simulink model "updated_target_driver_2026"  (R2024b)
settings: Solver=VariableStepAuto  StartTime=0.0  StopTime=10.0  RelTol=1e-3
values from neighbouring files (symbols this model uses):
  A = gamma_2*gamma_3*Thrust_desired    [force2voltage.m]
  a2_lb = -0.25    [target_driver_setup_2022_Ctrl_V_2_4.m]    (also in target_driver_setup_2022_Ctrl_V_2_4_geometric.m; target_driver_setup_mpc_12msdelay.m; target_driver_setup_mpc_andWLQP.m)
  a2_openloop = -0    (= 0)    [target_driver_setup_2022_Ctrl_V_2_4.m]    (also in target_driver_setup_2022_Ctrl_V_2_4_geometric.m; target_driver_setup_mpc_12msdelay.m; target_driver_setup_mpc_andWLQP.m)
  a2_ub = 0.25    [target_driver_setup_2022_Ctrl_V_2_4.m]    (also in target_driver_setup_2022_Ctrl_V_2_4_geometric.m; target_driver_setup_mpc_12msdelay.m; target_driver_setup_mpc_andWLQP.m)
  adaptive_flag = 0    [target_driver_setup_2022_Ctrl_V_2_4.m]    (also in target_driver_setup_2022_Ctrl_V_2_4_geometric.m; target_driver_setup_mpc_12msdelay.m = 1; target_driver_setup_mpc_andWLQP.m = 1)
  adaptive_gain = [gamma_adaptive, adaptive_roll_limit, adaptive_pitch_limit, adaptive_yaw_limit, c_2_adaptive, gamma_lateral_adaptive, adaptive_x_limit, adaptive_y_limit, adaptive_z_limit, c_1_adaptive]    [target_driver_setup_2022_Ctrl_V_2_4.m]    (also in target_driver_setup_2022_Ctrl_V_2_4_geometric.m; target_driver_setup_mpc_12msdelay.m; target_driver_setup_mpc_andWLQP.m)
  adaptive_lateral_flag = 0    [target_driver_setup_2022_Ctrl_V_2_4.m]    (also in target_driver_setup_2022_Ctrl_V_2_4_geometric.m; target_driver_setup_mpc_12msdelay.m = 1; target_driver_setup_mpc_andWLQP.m = 1)
  adaptive_pitch_init = 0    [target_driver_setup_2022_Ctrl_V_2_4.m]    (also in target_driver_setup_2022_Ctrl_V_2_4_geometric.m; target_driver_setup_mpc_12msdelay.m; target_driver_setup_mpc_andWLQP.m)
  adaptive_pitch_limit = 0.1/(scale^2)    (= 1e-07)    [target_driver_setup_2022_Ctrl_V_2_4.m]    (also in target_driver_setup_2022_Ctrl_V_2_4_geometric.m = 3e-07; target_driver_setup_mpc_12msdelay.m; target_driver_setup_mpc_andWLQP.m)
  adaptive_pitch_limit_low = -adaptive_pitch_limit    (= -1e-07)    [target_driver_setup_2022_Ctrl_V_2_4.m]    (also in target_driver_setup_2022_Ctrl_V_2_4_geometric.m = -3e-07; target_driver_setup_mpc_12msdelay.m; target_driver_setup_mpc_andWLQP.m)
  adaptive_roll_init = 0    [target_driver_setup_2022_Ctrl_V_2_4.m]    (also in target_driver_setup_2022_Ctrl_V_2_4_geometric.m; target_driver_setup_mpc_12msdelay.m; target_driver_setup_mpc_andWLQP.m)
  adaptive_roll_limit = 0.3/(scale^2)    (= 3e-07)    [target_driver_setup_2022_Ctrl_V_2_4.m]    (also in target_driver_setup_2022_Ctrl_V_2_4_geometric.m; target_driver_setup_mpc_12msdelay.m; target_driver_setup_mpc_andWLQP.m)
  adaptive_roll_limit_low = -adaptive_roll_limit    (= -3e-07)    [target_driver_setup_2022_Ctrl_V_2_4.m]    (also in target_driver_setup_2022_Ctrl_V_2_4_geometric.m; target_driver_setup_mpc_12msdelay.m; target_driver_setup_mpc_andWLQP.m)
  adaptive_x_init = 0    [target_driver_setup_2022_Ctrl_V_2_4.m]    (also in target_driver_setup_2022_Ctrl_V_2_4_geometric.m; target_driver_setup_mpc_12msdelay.m; target_driver_setup_mpc_andWLQP.m)
  adaptive_x_limit = 0.15/(scale)    (= 0.00015)    [target_driver_setup_2022_Ctrl_V_2_4.m]    (also in target_driver_setup_2022_Ctrl_V_2_4_geometric.m = 7.5e-05; target_driver_setup_mpc_12msdelay.m; target_driver_setup_mpc_andWLQP.m)
  adaptive_x_limit_low = -adaptive_x_limit    (= -0.00015)    [target_driver_setup_2022_Ctrl_V_2_4.m]    (also in target_driver_setup_2022_Ctrl_V_2_4_geometric.m = -7.5e-05; target_driver_setup_mpc_12msdelay.m; target_driver_setup_mpc_andWLQP.m)
  adaptive_y_init = 0    [target_driver_setup_2022_Ctrl_V_2_4.m]    (also in target_driver_setup_2022_Ctrl_V_2_4_geometric.m; target_driver_setup_mpc_12msdelay.m; target_driver_setup_mpc_andWLQP.m)
  adaptive_y_limit = 0.15/(scale)    (= 0.00015)    [target_driver_setup_2022_Ctrl_V_2_4.m]    (also in target_driver_setup_2022_Ctrl_V_2_4_geometric.m = 7.5e-05; target_driver_setup_mpc_12msdelay.m; target_driver_setup_mpc_andWLQP.m)
  adaptive_y_limit_low = -adaptive_y_limit    (= -0.00015)    [target_driver_setup_2022_Ctrl_V_2_4.m]    (also in target_driver_setup_2022_Ctrl_V_2_4_geometric.m = -7.5e-05; target_driver_setup_mpc_12msdelay.m; target_driver_setup_mpc_andWLQP.m)
  adaptive_yaw_init = 0    [target_driver_setup_2022_Ctrl_V_2_4.m]    (also in target_driver_setup_2022_Ctrl_V_2_4_geometric.m; target_driver_setup_mpc_12msdelay.m; target_driver_setup_mpc_andWLQP.m)
  adaptive_yaw_limit = 0.035/(scale^2)    (= 3.5e-08)    [target_driver_setup_2022_Ctrl_V_2_4.m]    (also in target_driver_setup_2022_Ctrl_V_2_4_geometric.m; target_driver_setup_mpc_12msdelay.m; target_driver_setup_mpc_andWLQP.m)
  adaptive_yaw_limit_low = -adaptive_yaw_limit    (= -3.5e-08)    [target_driver_setup_2022_Ctrl_V_2_4.m]    (also in target_driver_setup_2022_Ctrl_V_2_4_geometric.m; target_driver_setup_mpc_12msdelay.m; target_driver_setup_mpc_andWLQP.m)
  adaptive_z_init = 0/scale    (= 0)    [target_driver_setup_2022_Ctrl_V_2_4.m]    (also in target_driver_setup_2022_Ctrl_V_2_4_geometric.m; target_driver_setup_mpc_12msdelay.m; target_driver_setup_mpc_andWLQP.m)
  adaptive_z_limit = 0.20/(scale)    (= 0.0002)    [target_driver_setup_2022_Ctrl_V_2_4.m]    (also in target_driver_setup_2022_Ctrl_V_2_4_geometric.m = 0.0008; target_driver_setup_mpc_12msdelay.m = 0.0008; target_driver_setup_mpc_andWLQP.m = 0.0008)
  adaptive_z_limit_low = -adaptive_z_limit/1    (= -0.0002)    [target_driver_setup_2022_Ctrl_V_2_4.m]    (also in target_driver_setup_2022_Ctrl_V_2_4_geometric.m = -0.0008; target_driver_setup_mpc_12msdelay.m = -0.0008; target_driver_setup_mpc_andWLQP.m = -0.0008)
  att_s = 500    [target_driver_setup_2022_Ctrl_V_2_4.m]    (also in target_driver_setup_2022_Ctrl_V_2_4_geometric.m; target_driver_setup_mpc_12msdelay.m; target_driver_setup_mpc_andWLQP.m)
  b_1_d_desired = [1,0,0]    [target_driver_setup_2022_Ctrl_V_2_4.m]    (also in target_driver_setup_2022_Ctrl_V_2_4_geometric.m; target_driver_setup_mpc_12msdelay.m; target_driver_setup_mpc_andWLQP.m)
  closedloop_flag = 1    [target_driver_setup_2022_Ctrl_V_2_4.m]    (also in target_driver_setup_2022_Ctrl_V_2_4_geometric.m = 0; target_driver_setup_mpc_12msdelay.m = 0; target_driver_setup_mpc_andWLQP.m = 0)
  control_gain = [k_x,k_v, k_R, k_Omega, k_z, k_vz, k_Rx]    [target_driver_setup_2022_Ctrl_V_2_4.m]    (also in target_driver_setup_2022_Ctrl_V_2_4_geometric.m = [k_x,k_v,k_R,k_Omega_pitch,k_Omega_roll,k_z,k_vz,k_Rx]; target_driver_setup_mpc_12msdelay.m = [k_x, k_v, k_R, k_Omega, k_z, k_vz, k_Rx,                  k; target_driver_setup_mpc_andWLQP.m = [k_x, k_v, k_R, k_Omega, k_z, k_vz, k_Rx,                  k)
  delay = delay-vicon_sample_cycle/2    [target_driver_setup_2022_Ctrl_V_2_4.m]    (also in target_driver_setup_2022_Ctrl_V_2_4_geometric.m; target_driver_setup_mpc_12msdelay.m; target_driver_setup_mpc_andWLQP.m)
  drv_amp = abs((vleft_p2p-vright_p2p))/2+min(vleft_p2p,vright_p2p)    [Wing_traj_to_Voltage.m]    (also in force2voltage.m; target_driver_setup_2022_Ctrl_V_2_4.m = 300; target_driver_setup_2022_Ctrl_V_2_4_geometric.m = 110; target_driver_setup_mpc_12msdelay.m = 150)
  drv_bias = max_drv_bias    (= 300)    [target_driver_setup_2022_Ctrl_V_2_4.m]    (also in target_driver_setup_2022_Ctrl_V_2_4_geometric.m = 200; target_driver_setup_mpc_12msdelay.m = 200; target_driver_setup_mpc_andWLQP.m = 200)
  drv_pitch_left = vleft_pitch    [Wing_traj_to_Voltage.m]    (also in force2voltage.m = 0; target_driver_setup_2022_Ctrl_V_2_4.m = 0; target_driver_setup_2022_Ctrl_V_2_4_geometric.m = 9.05; target_driver_setup_mpc_12msdelay.m = 9.05)
  drv_pitch_right = vright_pitch    [Wing_traj_to_Voltage.m]    (also in force2voltage.m = 0; target_driver_setup_2022_Ctrl_V_2_4.m = 0; target_driver_setup_2022_Ctrl_V_2_4_geometric.m = 9.05; target_driver_setup_mpc_12msdelay.m = 9.05)
  drv_roll = (vleft_p2p-vright_p2p)/4    [Wing_traj_to_Voltage.m]    (also in force2voltage.m; target_driver_setup_2022_Ctrl_V_2_4.m = 0; target_driver_setup_2022_Ctrl_V_2_4_geometric.m = -0.001; target_driver_setup_mpc_12msdelay.m = -0.001)
  f_fin = f    (= 180)    [target_driver_setup_2022_Ctrl_V_2_4.m]    (also in target_driver_setup_2022_Ctrl_V_2_4_geometric.m = 155; target_driver_setup_mpc_12msdelay.m = 155; target_driver_setup_mpc_andWLQP.m = 155)
  f_int = f    (= 180)    [target_driver_setup_2022_Ctrl_V_2_4.m]    (also in target_driver_setup_2022_Ctrl_V_2_4_geometric.m = 155; target_driver_setup_mpc_12msdelay.m = 155; target_driver_setup_mpc_andWLQP.m = 155)
  g = 9.8    [target_driver_setup_2022_Ctrl_V_2_4.m]    (also in target_driver_setup_2022_Ctrl_V_2_4_geometric.m; target_driver_setup_mpc_12msdelay.m; target_driver_setup_mpc_andWLQP.m = 9.81; test_full_attitude_mpc.m = 9.81)
  I_moment_vec = [Ixx, Iyy, Izz]    [target_driver_setup_2022_Ctrl_V_2_4.m]    (also in target_driver_setup_2022_Ctrl_V_2_4_geometric.m; target_driver_setup_mpc_12msdelay.m; target_driver_setup_mpc_andWLQP.m)
  landing_flag = 0    [target_driver_setup_2022_Ctrl_V_2_4.m]    (also in target_driver_setup_2022_Ctrl_V_2_4_geometric.m; target_driver_setup_mpc_12msdelay.m; target_driver_setup_mpc_andWLQP.m)
  landing_parameter = [start_delay+T,transition_rate, rising_time, falling_time, landing_rising_time, landing_z_decrease, landing_y_decrease, landing_x_decrease]    [target_driver_setup_2022_Ctrl_V_2_4.m]    (also in target_driver_setup_2022_Ctrl_V_2_4_geometric.m; target_driver_setup_mpc_12msdelay.m; target_driver_setup_mpc_andWLQP.m)
  low_bound = -8    [target_driver_setup_2022_Ctrl_V_2_4.m]    (also in target_driver_setup_2022_Ctrl_V_2_4_geometric.m = -5; target_driver_setup_mpc_12msdelay.m = -10; target_driver_setup_mpc_andWLQP.m = -10)
  low_bound_eR = -0.8    [target_driver_setup_2022_Ctrl_V_2_4.m]    (also in target_driver_setup_2022_Ctrl_V_2_4_geometric.m = -1.2; target_driver_setup_mpc_12msdelay.m = -1.2; target_driver_setup_mpc_andWLQP.m = -1.2)
  low_bound_vx = -0.5    [target_driver_setup_2022_Ctrl_V_2_4.m]    (also in target_driver_setup_2022_Ctrl_V_2_4_geometric.m; target_driver_setup_mpc_12msdelay.m; target_driver_setup_mpc_andWLQP.m)
  low_bound_vy = -0.5    [target_driver_setup_2022_Ctrl_V_2_4.m]    (also in target_driver_setup_2022_Ctrl_V_2_4_geometric.m; target_driver_setup_mpc_12msdelay.m; target_driver_setup_mpc_andWLQP.m)
  low_bound_vz = -0.5    [target_driver_setup_2022_Ctrl_V_2_4.m]    (also in target_driver_setup_2022_Ctrl_V_2_4_geometric.m; target_driver_setup_mpc_12msdelay.m; target_driver_setup_mpc_andWLQP.m)
  low_bound_x = -0.06    [target_driver_setup_2022_Ctrl_V_2_4.m]    (also in target_driver_setup_2022_Ctrl_V_2_4_geometric.m = -0.1; target_driver_setup_mpc_12msdelay.m = -0.6; target_driver_setup_mpc_andWLQP.m = -0.6)
  low_bound_y = -0.06    [target_driver_setup_2022_Ctrl_V_2_4.m]    (also in target_driver_setup_2022_Ctrl_V_2_4_geometric.m; target_driver_setup_mpc_12msdelay.m = -0.6; target_driver_setup_mpc_andWLQP.m = -0.6)
  low_bound_z = -0.04    [target_driver_setup_2022_Ctrl_V_2_4.m]    (also in target_driver_setup_2022_Ctrl_V_2_4_geometric.m; target_driver_setup_mpc_12msdelay.m = -0.1; target_driver_setup_mpc_andWLQP.m = -0.1)
  m = t <= t_zoom    [plot_roll_torque_cmd_vs_actual.m]    (also in plot_roll_torque_cmd_vs_actual_flightlog.m = t >= t0 & t <= t1; target_driver_setup_2022_Ctrl_V_2_4.m = 0.000124; target_driver_setup_2022_Ctrl_V_2_4_geometric.m = 8.5655e-05; target_driver_setup_mpc_12msdelay.m = 8.5655e-05)
  params_vec = [params_opt.delta_1, params_opt.delta_2, params_opt.delta_3,      params_opt.gamma_1, params_opt.gamma_2_1, params_opt.gamma_3,      params_opt.eta, params_opt.nu, params_opt.mu]'    [force2voltage_tuningSandbox.m]    (also in target_driver_setup_2022_Ctrl_V_2_4.m = [params_opt.delta_1, params_opt.delta_2, params_opt.delta_3,; target_driver_setup_2022_Ctrl_V_2_4_geometric.m = [params_opt.delta_1, params_opt.delta_2, params_opt.delta_3,; target_driver_setup_mpc_12msdelay.m = [params_opt.delta_1, params_opt.delta_2, params_opt.delta_3,; target_driver_setup_mpc_andWLQP.m = [params_opt.delta_1, params_opt.delta_2, params_opt.delta_3,)
  phase = 0    [target_driver_setup_2022_Ctrl_V_2_4.m]    (also in target_driver_setup_2022_Ctrl_V_2_4_geometric.m; target_driver_setup_mpc_12msdelay.m; target_driver_setup_mpc_andWLQP.m)
  r_desired = [default_x, default_y,z_desired]    [target_driver_setup_2022_Ctrl_V_2_4.m]    (also in target_driver_setup_2022_Ctrl_V_2_4_geometric.m; target_driver_setup_mpc_12msdelay.m; target_driver_setup_mpc_andWLQP.m)
  roll_offset_angle = 0    [target_driver_setup_2022_Ctrl_V_2_4.m]    (also in target_driver_setup_2022_Ctrl_V_2_4_geometric.m; target_driver_setup_mpc_12msdelay.m; target_driver_setup_mpc_andWLQP.m)
  running_time = start_delay+total_T    (= 9)    [target_driver_setup_2022_Ctrl_V_2_4.m]    (also in target_driver_setup_2022_Ctrl_V_2_4_geometric.m = 10; target_driver_setup_mpc_12msdelay.m = 0.5; target_driver_setup_mpc_andWLQP.m = 10)
  running_time_control = start_delay_control+total_T+0.0    (= 7.1)    [target_driver_setup_2022_Ctrl_V_2_4.m]    (also in target_driver_setup_2022_Ctrl_V_2_4_geometric.m = 10; target_driver_setup_mpc_12msdelay.m = 0.5; target_driver_setup_mpc_andWLQP.m = 10)
  start_delay = 2.0    (= 2)    [target_driver_setup_2022_Ctrl_V_2_4.m]    (also in target_driver_setup_2022_Ctrl_V_2_4_geometric.m = 0; target_driver_setup_mpc_12msdelay.m = 0; target_driver_setup_mpc_andWLQP.m = 0)
  start_delay_control = start_delay + ramp_delay    (= 0.1)    [target_driver_setup_2022_Ctrl_V_2_4.m]    (also in target_driver_setup_2022_Ctrl_V_2_4_geometric.m = 0; target_driver_setup_mpc_12msdelay.m = 0; target_driver_setup_mpc_andWLQP.m = 0)
  T = 1    [target_driver_setup_2022_Ctrl_V_2_4.m]    (also in target_driver_setup_2022_Ctrl_V_2_4_geometric.m = 10; target_driver_setup_mpc_12msdelay.m = 0.5; target_driver_setup_mpc_andWLQP.m = 10; test_full_attitude_mpc.m = T0 + nu(1))
  task_flag = 0    [target_driver_setup_2022_Ctrl_V_2_4.m]    (also in target_driver_setup_2022_Ctrl_V_2_4_geometric.m; target_driver_setup_mpc_12msdelay.m; target_driver_setup_mpc_andWLQP.m)
  task_parameter = [radius_ref, frequency_ref, radius_ratio, lissajous_ratio, lissajous_delta, lissajous_amplitude_ratio,z_radius_ratio]    [target_driver_setup_2022_Ctrl_V_2_4.m]    (also in target_driver_setup_2022_Ctrl_V_2_4_geometric.m; target_driver_setup_mpc_12msdelay.m; target_driver_setup_mpc_andWLQP.m)
  upp_bound = 8    [target_driver_setup_2022_Ctrl_V_2_4.m]    (also in target_driver_setup_2022_Ctrl_V_2_4_geometric.m = 5; target_driver_setup_mpc_12msdelay.m = 10; target_driver_setup_mpc_andWLQP.m = 10)
  upp_bound_eR = 0.8    [target_driver_setup_2022_Ctrl_V_2_4.m]    (also in target_driver_setup_2022_Ctrl_V_2_4_geometric.m = 1.2; target_driver_setup_mpc_12msdelay.m = 1.2; target_driver_setup_mpc_andWLQP.m = 1.2)
  upp_bound_vx = 0.5    [target_driver_setup_2022_Ctrl_V_2_4.m]    (also in target_driver_setup_2022_Ctrl_V_2_4_geometric.m; target_driver_setup_mpc_12msdelay.m; target_driver_setup_mpc_andWLQP.m)
  upp_bound_vy = 0.5    [target_driver_setup_2022_Ctrl_V_2_4.m]    (also in target_driver_setup_2022_Ctrl_V_2_4_geometric.m; target_driver_setup_mpc_12msdelay.m; target_driver_setup_mpc_andWLQP.m)
  upp_bound_vz = 0.5    [target_driver_setup_2022_Ctrl_V_2_4.m]    (also in target_driver_setup_2022_Ctrl_V_2_4_geometric.m; target_driver_setup_mpc_12msdelay.m; target_driver_setup_mpc_andWLQP.m)
  upp_bound_x = 0.06    [target_driver_setup_2022_Ctrl_V_2_4.m]    (also in target_driver_setup_2022_Ctrl_V_2_4_geometric.m = 0.1; target_driver_setup_mpc_12msdelay.m = 0.6; target_driver_setup_mpc_andWLQP.m = 0.6)
  upp_bound_y = 0.06    [target_driver_setup_2022_Ctrl_V_2_4.m]    (also in target_driver_setup_2022_Ctrl_V_2_4_geometric.m; target_driver_setup_mpc_12msdelay.m = 0.6; target_driver_setup_mpc_andWLQP.m = 0.6)
  upp_bound_z = 0.04    [target_driver_setup_2022_Ctrl_V_2_4.m]    (also in target_driver_setup_2022_Ctrl_V_2_4_geometric.m; target_driver_setup_mpc_12msdelay.m = 0.1; target_driver_setup_mpc_andWLQP.m = 0.1)
undefined symbols (not defined in the file or in its folder): Com1, DiscIntNeverNeededParam, dspblkCoreblockFVToolHelper, gcbh, left_mapping, left_mapping_F_to_Phi, lp_den, lp_num, none, right_mapping, right_mapping_F_to_Phi, vlp_den, vlp_num
libraries: simulink x25, xpcseriallib x4, xpcnilib x2, xpcutilitieslib x2
(part 2 of 6)

== system updated_target_driver_2026/Geometric Controller/lateral adaptive ==
  e_x : Inport
  e_v : Inport  Port=2
  Enable : Inport  Port=3
  adaptive_gain : Inport  Port=4
  Adaptive_lateral_flag : Inport  Port=5
  Adaptive Control : MATLAB Function  TreatAsAtomicUnit=on
  Compare To Zero : simulink/Logic and Bit Operations/Compare To Zero  relop=>  OutDataTypeStr=uint8  ZeroCross=off
  "Integrator " : DiscreteIntegrator  InitialConditionSource=external  InitialCondition=adaptive_roll_init  SampleTime=-1  LimitOutput=on  UpperSaturationLimit=adaptive_x_limit  LowerSaturationLimit=adaptive_x_limit_low  ICPrevOutput=DiscIntNeverNeededParam  ICPrevScaledInput=DiscIntNeverNeededParam
  Integrator 1 : DiscreteIntegrator  InitialConditionSource=external  InitialCondition=adaptive_pitch_init  SampleTime=-1  LimitOutput=on  UpperSaturationLimit=adaptive_y_limit  LowerSaturationLimit=adaptive_y_limit_low  ICPrevOutput=DiscIntNeverNeededParam  ICPrevScaledInput=DiscIntNeverNeededParam
  Integrator 2 : DiscreteIntegrator  InitialConditionSource=external  InitialCondition=adaptive_yaw_init  SampleTime=-1  LimitOutput=on  UpperSaturationLimit=adaptive_z_limit  LowerSaturationLimit=adaptive_z_limit_low  ICPrevOutput=DiscIntNeverNeededParam  ICPrevScaledInput=DiscIntNeverNeededParam
  Mux : Mux  Inputs=3
  Product{1,5..10} (7 alike) : Product  RndMeth=Zero
  "adaptive_x_init " : Constant  Value=adaptive_x_init
  adaptive_y_init : Constant  Value=adaptive_y_init
  adaptive_z_init : Constant  Value=adaptive_z_init
  adaptive_lateral_control : Outport
  adaptive_x : Outport  Port=2
  adaptive_y : Outport  Port=3
  adaptive_z : Outport  Port=4
  wires:
  Product5/1 -> "Integrator "/1
  Adaptive Control/1(der_adaptive_torque_x) -> Product5/2
  Product6/1 -> Integrator 1/1
  Adaptive Control/2(der_adaptive_torque_y) -> Product6/2
  Product7/1 -> Integrator 2/1
  Adaptive Control/3(der_adaptive_torque_z) -> Product7/2
  adaptive_gain/1 -> Adaptive Control/6(adaptive_gain_limit)
  "adaptive_x_init "/1 -> "Integrator "/2
  adaptive_y_init/1 -> Integrator 1/2
  adaptive_z_init/1 -> Integrator 2/2
  e_x/1 -> Adaptive Control/4(e_x)
  Enable/1 -> Product7/1, Product6/1, Product5/1
  e_v/1 -> Adaptive Control/5(e_v)
  Compare To Zero/1 -> Product1/1, Product10/1, Product9/1, Product8/1
  Adaptive_lateral_flag/1 -> Compare To Zero/1
  "Integrator "/1 -> Adaptive Control/1(current_adaptive_x), Product8/2, Mux/1
  Integrator 1/1 -> Adaptive Control/2(current_adaptive_y), Product9/2, Mux/2
  Product9/1 -> adaptive_y/1
  Product8/1 -> adaptive_x/1
  Integrator 2/1 -> Product10/2, Mux/3, Adaptive Control/3(current_adaptive_z)
  Product10/1 -> adaptive_z/1
  Mux/1 -> Product1/2
  Product1/1 -> adaptive_lateral_control/1

== system updated_target_driver_2026/Observer for averaged system1/Attitude Observer ==
  note: Attitude averaging and filtering using geometric average in Riemannian metric SO(3)
      |
      | Patrick 2021 Mar
  Vicon Update flag : Inport
  Raw Rotation : Inport  Port=2
  Vicon Count : Inport  Port=3
  Geometric Averaging Rotation Matix : Subsystem
  Geometric derivative in SO(3) : Subsystem
  "Averaged quaternion " : Outport
  Average Rotation Matrix : Outport  Port=2
  Raw quaternion : Outport  Port=3
  Geometric filtered derivative : Outport  Port=4
  wires:
  Vicon Count/1 -> Geometric derivative in SO(3)/2(Vicon Count)
  Raw Rotation/1 -> Geometric Averaging Rotation Matix/2(Current Rotation)
  Vicon Update flag/1 -> Geometric derivative in SO(3)/4("Vicon Update Flag "), Geometric Averaging Rotation Matix/1(Vicon Update flag)
  Geometric Averaging Rotation Matix/4(Previous Averaged Rotation Matrix) -> Geometric derivative in SO(3)/1(Previous Averaged Rotation M)
  Geometric derivative in SO(3)/1(Filtered Geometric derivative in SO(3)) -> Geometric filtered derivative/1
  Geometric Averaging Rotation Matix/3("Raw quaternion output ") -> Raw quaternion/1
  Geometric Averaging Rotation Matix/1(Averaged quaternion output) -> "Averaged quaternion "/1
  Geometric Averaging Rotation Matix/2("Averaged Rotation Matrix ") -> Average Rotation Matrix/1, Geometric derivative in SO(3)/3(Current Averaged Rotation M)

== system updated_target_driver_2026/Observer for averaged system1/Euler derivative & filtered angular velocity  ==
  note: The skew symmetric structure is corrected from
      | the old angular velocity calculation.
      | Note from Patrick 2021 Mar
  "Rotation matrix " : Inport
  Angular velocity : MATLAB Function  TreatAsAtomicUnit=on
  Demux : Demux  Outputs=3
  Mux : Mux  Inputs=3
  filtered derivative : Subsystem
  Angular velocity_Euler : Outport
  Frob_norm error : Outport  Port=2
  wires:
  Demux/2 -> Mux/2
  Demux/3 -> Mux/3
  Mux/1 -> Angular velocity_Euler/1
  filtered derivative/1(Out1) -> Angular velocity/2(Rdot)
  Angular velocity/1(w) -> Demux/1
  Demux/1 -> Mux/1
  Angular velocity/2(Frob_error) -> Frob_norm error/1
  "Rotation matrix "/1 -> Angular velocity/1(R), filtered derivative/1(In1)

== system updated_target_driver_2026/Observer for averaged system1/Position Observer ==
  "raw_position " : Inport
  vicon Update : Inport  Port=2
  Vicon Count : Inport  Port=3
  "Averaging position & velocity " : MATLAB Function  TreatAsAtomicUnit=on
  Delay10 : Delay  DelayLength=delay(2)  InitialCondition=0
  Delay11 : Delay  DelayLength=delay(3)  InitialCondition=0
  Delay14 : Delay  DelayLength=delay(4)  InitialCondition=0
  LowPassFiltere1 : Subsystem
  LowPassFiltere2 : Subsystem
  previous position : Delay  DelayLength=1  InitialCondition=0
  previous velocity : Delay  DelayLength=1  InitialCondition=0
  Average and filtered position : Outport
  Averaged and filtered velocity : Outport  Port=2
  wires:
  previous velocity/1 -> "Averaging position & velocity "/8(vout_prev)
  "Averaging position & velocity "/2(vout) -> previous velocity/1, LowPassFiltere2/1(In1)
  previous position/1 -> "Averaging position & velocity "/7(rout_prev)
  "raw_position "/1 -> "Averaging position & velocity "/4(r_cur), Delay14/1, Delay11/1, Delay10/1
  Delay14/1 -> "Averaging position & velocity "/3(r_prev3)
  Delay11/1 -> "Averaging position & velocity "/2(r_prev2)
  Delay10/1 -> "Averaging position & velocity "/1(r_prev)
  LowPassFiltere2/1(Out1) -> Averaged and filtered velocity/1
  "Averaging position & velocity "/1(rout) -> previous position/1, LowPassFiltere1/1(In1)
  LowPassFiltere1/1(Out1) -> Average and filtered position/1
  vicon Update/1 -> "Averaging position & velocity "/5(update)
  Vicon Count/1 -> "Averaging position & velocity "/6(count)

== system updated_target_driver_2026/Open_Closed_loop_selection/SIgnalForRamp_binary ==
  note: Should output 1 or -1,
      | so signal ramps UP to 1
      | or DOWN to 0.
  In1 : Inport
  Add : Sum  Inputs=+-
  Compare To Zero : simulink/Logic and Bit Operations/Compare To Zero  relop=>  OutDataTypeStr=uint8  ZeroCross=off
  Constant : Constant
  Data Type Conversion : DataTypeConversion  OutDataTypeStr=double  SaturateOnIntegerOverflow=off  RndMeth=Floor
  Gain : Gain  Gain=2
  Out1 : Outport
  wires:
  In1/1 -> Compare To Zero/1
  Compare To Zero/1 -> Data Type Conversion/1
  Gain/1 -> Add/1
  Constant/1 -> Add/2
  Add/1 -> Out1/1
  Data Type Conversion/1 -> Gain/1

== system updated_target_driver_2026/Open_Closed_loop_selection/counter ==
  running time : Inport
  Add : Sum  Inputs=+-
  Compare To Zero : simulink/Logic and Bit Operations/Compare To Zero  relop=<  OutDataTypeStr=uint8  ZeroCross=off
  Product2 : Product  RndMeth=Zero
  SaturatingRamp : DiscreteIntegrator  gainval=1  SampleTime=-1  UpperSaturationLimit=1  LowerSaturationLimit=0  ICPrevOutput=DiscIntNeverNeededParam  ICPrevScaledInput=DiscIntNeverNeededParam
  constant : Constant
  start delay compare : simulink/Logic and Bit Operations/Compare To Constant  relop=>  const=start_delay  OutDataTypeStr=uint8
  enable : Outport
  wires:
  SaturatingRamp/1 -> Add/1, start delay compare/1
  running time/1 -> Add/2
  Add/1 -> Compare To Zero/1
  start delay compare/1 -> Product2/1
  Compare To Zero/1 -> Product2/2
  Product2/1 -> enable/1
  constant/1 -> SaturatingRamp/1

== system updated_target_driver_2026/Open_Closed_loop_selection/counter1 ==
  running time : Inport
  Add : Sum  Inputs=+-
  Compare To Zero : simulink/Logic and Bit Operations/Compare To Zero  relop=<  OutDataTypeStr=uint8  ZeroCross=off
  Product2 : Product  RndMeth=Zero
  SaturatingRamp : DiscreteIntegrator  gainval=1  SampleTime=-1  UpperSaturationLimit=1  LowerSaturationLimit=0  ICPrevOutput=DiscIntNeverNeededParam  ICPrevScaledInput=DiscIntNeverNeededParam
  constant : Constant
  start control delay compare : simulink/Logic and Bit Operations/Compare To Constant  relop=>  const=start_delay_control  OutDataTypeStr=uint8
  enable : Outport
  wires:
  SaturatingRamp/1 -> Add/1, start control delay compare/1
  running time/1 -> Add/2
  Add/1 -> Compare To Zero/1
  start control delay compare/1 -> Product2/1
  Compare To Zero/1 -> Product2/2
  Product2/1 -> enable/1
  constant/1 -> SaturatingRamp/1

== system updated_target_driver_2026/Open_Closed_loop_selection/timer1 ==
  SaturatingRamp : DiscreteIntegrator  gainval=1  SampleTime=-1  UpperSaturationLimit=1  LowerSaturationLimit=0  ICPrevOutput=DiscIntNeverNeededParam  ICPrevScaledInput=DiscIntNeverNeededParam
  constant : Constant
  time : Outport
  wires:
  SaturatingRamp/1 -> time/1
  constant/1 -> SaturatingRamp/1

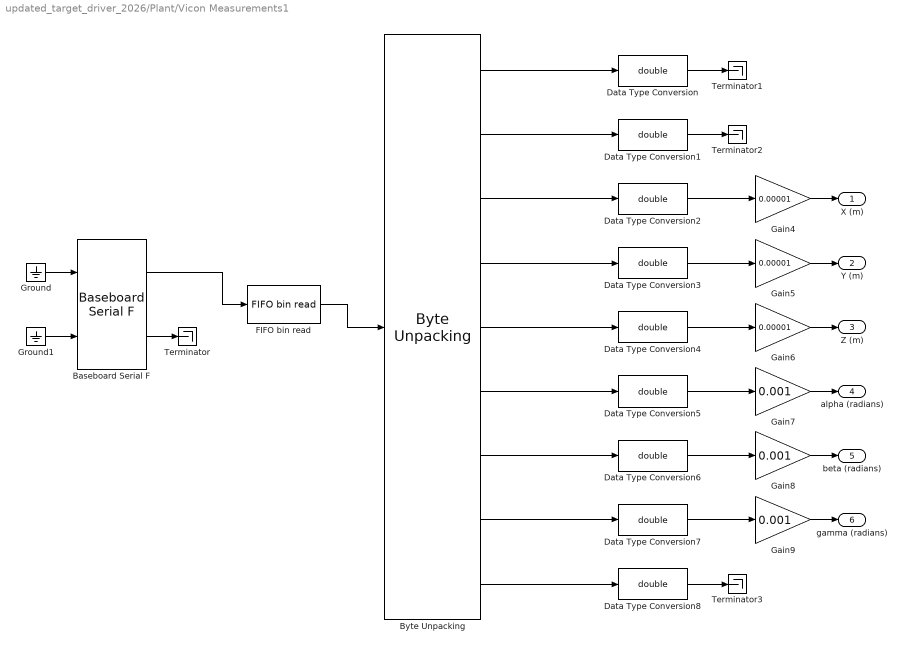
== system updated_target_driver_2026/Plant/Vicon Measurements1 ==
  Baseboard Serial F : xpcseriallib/Mainboard/Baseboard Serial F  group=FIFO Setup  port=1  irqnum=4  saddr1=0x3f8  saddr2=0x3e8  config=Com1/none  baud1=115200  parity1=None  ndata1=8  nstop1=1  fifomode1=16 deep  rlevel1=half full  automode1=on  xmtfifosize1=1024  xmtdatatype1=8 bit int null terminated  rcvfifosize1=1024  baud2=115200  parity2=None  ndata2=8  nstop2=1  fifomode2=16 deep  rlevel2=half full  automode2=off  xmtfifosize2=1024  xmtdatatype2=8 bit uint null terminated  rcvfifosize2=1024
      settings: SourceProductName=Simulink Real-Time
  "Byte Unpacking " : xpcutilitieslib/Byte Unpacking   MaskUnpackedDataTypes={'uint8','int16','int16','int16','int16','int16','int16','int16','uint8'}  MaskUnpackedDataSizes={[1] [1] [1] [1] [1] [1] [1] [1] [1]}  MaskAlignment=1
      settings: SourceProductName=Simulink Real-Time
  Data Type Conversion{,1..8} (9 alike) : DataTypeConversion  OutDataTypeStr=double  SaturateOnIntegerOverflow=off  RndMeth=Floor
  "FIFO bin read " : xpcseriallib/FIFO bin read   header=[128,127,127]  lengths=[15]  hold=Hold last output if no new data  enable=off  maxsize=15  outputtype=8 bit uint null terminated  sampletime=0.0001
      settings: SourceProductName=Simulink Real-Time
  Gain4 : Gain  Gain=0.00001
  Gain5 : Gain  Gain=0.00001
  Gain6 : Gain  Gain=0.00001
  Gain7 : Gain  Gain=0.001
  Gain8 : Gain  Gain=0.001
  Gain9 : Gain  Gain=0.001
  Ground : Ground
  Ground1 : Ground
  Terminator{,1..3} (4 alike) : Terminator
  X (m) : Outport
  Y (m) : Outport  Port=2
  Z (m) : Outport  Port=3
  alpha (radians) : Outport  Port=4
  beta (radians) : Outport  Port=5
  gamma (radians) : Outport  Port=6
  wires:
  Baseboard Serial F/1 -> "FIFO bin read "/1
  Baseboard Serial F/2 -> Terminator/1
  Ground1/1 -> Baseboard Serial F/2
  Ground/1 -> Baseboard Serial F/1
  "Byte Unpacking "/1 -> Data Type Conversion/1
  "Byte Unpacking "/2 -> Data Type Conversion1/1
  "Byte Unpacking "/3 -> Data Type Conversion2/1
  "Byte Unpacking "/4 -> Data Type Conversion3/1
  "FIFO bin read "/1 -> "Byte Unpacking "/1
  "Byte Unpacking "/8 -> Data Type Conversion7/1
  "Byte Unpacking "/7 -> Data Type Conversion6/1
  "Byte Unpacking "/5 -> Data Type Conversion4/1
  "Byte Unpacking "/6 -> Data Type Conversion5/1
  Data Type Conversion3/1 -> Gain5/1
  Data Type Conversion4/1 -> Gain6/1
  Data Type Conversion5/1 -> Gain7/1
  Data Type Conversion6/1 -> Gain8/1
  Data Type Conversion7/1 -> Gain9/1
  "Byte Unpacking "/9 -> Data Type Conversion8/1
  Gain4/1 -> X (m)/1
  Data Type Conversion2/1 -> Gain4/1
  Gain5/1 -> Y (m)/1
  Gain6/1 -> Z (m)/1
  Gain7/1 -> alpha (radians)/1
  Gain8/1 -> beta (radians)/1
  Gain9/1 -> gamma (radians)/1
  Data Type Conversion/1 -> Terminator1/1
  Data Type Conversion1/1 -> Terminator2/1
  Data Type Conversion8/1 -> Terminator3/1

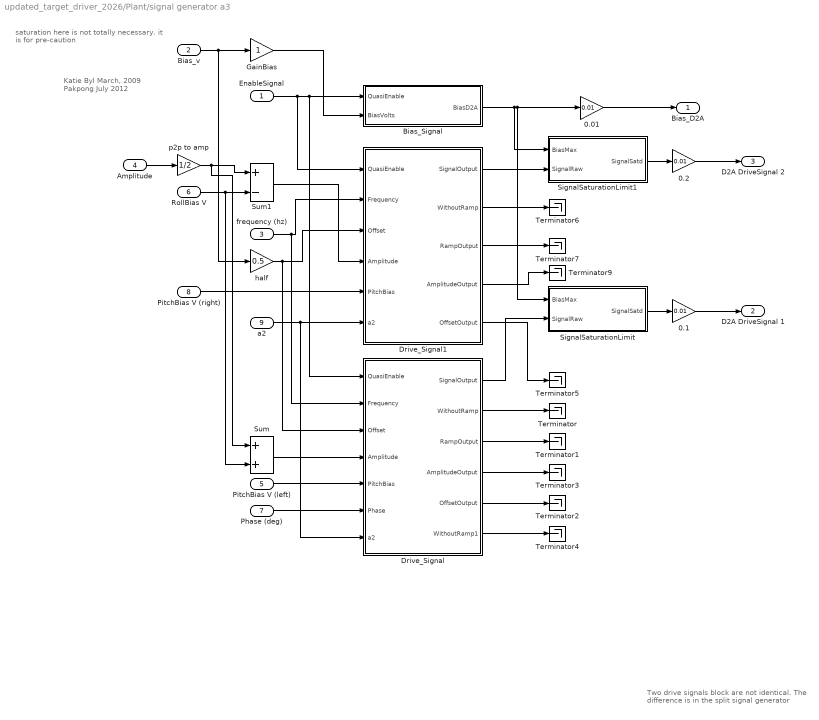
== system updated_target_driver_2026/Plant/signal generator a3 ==
  note: Katie Byl
      | March, 2009
      |
      | Pakpong
      | July 2012
  note: Two drive signals block are not identical.
      | The difference is in the split signal generator
  note: saturation here is not totally necessary.
      | it is for pre-caution
  EnableSignal : Inport
  Bias_v : Inport  Port=2
  frequency (hz) : Inport  Port=3
  Amplitude : Inport  Port=4
  PitchBias V (left) : Inport  Port=5
  RollBias V : Inport  Port=6
  Phase (deg) : Inport  Port=7
  PitchBias V (right) : Inport  Port=8
  a2 : Inport  Port=9
  0.01 : Gain  Gain=0.01
  0.1 : Gain  Gain=0.01
  0.2 : Gain  Gain=0.01
  Bias_Signal : Subsystem
  Drive_Signal : Subsystem
  Drive_Signal1 : Subsystem
  GainBias : Gain
  SignalSaturationLimit : Subsystem
  SignalSaturationLimit1 : Subsystem
  Sum : Sum
  Sum1 : Sum  Inputs=+-
  Terminator{,1..7,9} (9 alike) : Terminator
  half : Gain  Gain=0.5
  p2p to amp : Gain  Gain=1/2
  Bias_D2A : Outport
  D2A DriveSignal 1 : Outport  Port=2
  D2A DriveSignal 2 : Outport  Port=3
  wires:
  0.1/1 -> D2A DriveSignal 1/1
  0.2/1 -> D2A DriveSignal 2/1
  SignalSaturationLimit1/1(SignalSatd) -> 0.2/1
  0.01/1 -> Bias_D2A/1
  SignalSaturationLimit/1(SignalSatd) -> 0.1/1
  Drive_Signal/5(OffsetOutput) -> Terminator2/1
  GainBias/1 -> Bias_Signal/2(BiasVolts)
  Drive_Signal/1(SignalOutput) -> SignalSaturationLimit/2(SignalRaw)
  Drive_Signal1/5(OffsetOutput) -> Terminator5/1
  half/1 -> Drive_Signal1/3(Offset), Drive_Signal/3(Offset)
  Drive_Signal1/4(AmplitudeOutput) -> Terminator9/1
  Drive_Signal1/3(RampOutput) -> Terminator7/1
  PitchBias V (left)/1 -> Drive_Signal/5(PitchBias)
  Bias_Signal/1(BiasD2A) -> 0.01/1, SignalSaturationLimit/1(BiasMax), SignalSaturationLimit1/1(BiasMax)
  Drive_Signal1/2(WithoutRamp) -> Terminator6/1
  Drive_Signal/6(WithoutRamp1) -> Terminator4/1
  a2/1 -> Drive_Signal1/6(a2), Drive_Signal/7("a2 ")
  Drive_Signal/2(WithoutRamp) -> Terminator/1
  Phase (deg)/1 -> Drive_Signal/6(Phase)
  frequency (hz)/1 -> Drive_Signal/2(Frequency), Drive_Signal1/2(Frequency)
  RollBias V/1 -> Sum1/2, Sum/2
  Sum1/1 -> Drive_Signal1/4(Amplitude)
  Drive_Signal/4(AmplitudeOutput) -> Terminator3/1
  PitchBias V (right)/1 -> Drive_Signal1/5(PitchBias)
  EnableSignal/1 -> Bias_Signal/1(QuasiEnable), Drive_Signal/1(QuasiEnable), Drive_Signal1/1(QuasiEnable)
  Amplitude/1 -> p2p to amp/1
  Sum/1 -> Drive_Signal/4(Amplitude)
  Bias_v/1 -> half/1, GainBias/1
  Drive_Signal/3(RampOutput) -> Terminator1/1
  Drive_Signal1/1(SignalOutput) -> SignalSaturationLimit1/2(SignalRaw)
  p2p to amp/1 -> Sum1/1, Sum/1

== system updated_target_driver_2026/Variant Subsystem/Plant ==
  EnableSignal : Inport
  frequency (hz) : Inport  Port=2
  Amplitude : Inport  Port=3
  PitchBias V (left) : Inport  Port=4
  RollBias V : Inport  Port=5
  PitchBias V (right) : Inport  Port=6
  a2 : Inport  Port=7
  Bias_v : Inport  Port=8
  Phase (deg) : Inport  Port=9
  In10 : Inport  Port=10
  PCI-6259 DA1 : xpcnilib/D//A/M Series/PCI-6259 DA  channel=[1:4]  range=[10,5, 10, 10]  reset=[1 1 1 1]  initValue=[0 0 0 0]  sampletime=-1  slot=-1
      settings: SourceProductName=Simulink Real-Time
  Vicon Measurements1 : Subsystem
  signal generator a3 : Subsystem
  bias2 : Outport
  LW signal2 : Outport  Port=2
  RW signal2 : Outport  Port=3
  X (m) : Outport  Port=4
  Y (m) : Outport  Port=5
  Z (m) : Outport  Port=6
  alpha (radians) : Outport  Port=7
  beta (radians) : Outport  Port=8
  gamma (radians) : Outport  Port=9
  wires:
  Vicon Measurements1/2(Y (m)) -> Y (m)/1
  PitchBias V (right)/1 -> signal generator a3/8(PitchBias V (right))
  a2/1 -> signal generator a3/9(a2)
  Phase (deg)/1 -> signal generator a3/7(Phase (deg))
  Vicon Measurements1/4(alpha (radians)) -> alpha (radians)/1
  frequency (hz)/1 -> signal generator a3/3(frequency (hz))
  RollBias V/1 -> signal generator a3/6(RollBias V)
  Bias_v/1 -> signal generator a3/2(Bias_v)
  Vicon Measurements1/6(gamma (radians)) -> gamma (radians)/1
  Amplitude/1 -> signal generator a3/4(Amplitude)
  Vicon Measurements1/5(beta (radians)) -> beta (radians)/1
  signal generator a3/3(D2A DriveSignal 2) -> RW signal2/1, PCI-6259 DA1/3
  signal generator a3/1(Bias_D2A) -> bias2/1, PCI-6259 DA1/1
  Vicon Measurements1/1(X (m)) -> X (m)/1
  Vicon Measurements1/3(Z (m)) -> Z (m)/1
  In10/1 -> PCI-6259 DA1/4
  PitchBias V (left)/1 -> signal generator a3/5(PitchBias V (left))
  EnableSignal/1 -> signal generator a3/1(EnableSignal)
  signal generator a3/2(D2A DriveSignal 1) -> LW signal2/1, PCI-6259 DA1/2

== system updated_target_driver_2026/Variant Subsystem/Subsystem ==
  EnableSignal : Inport
  frequency (hz) : Inport  Port=2
  Amplitude : Inport  Port=3
  PitchBias V (left) : Inport  Port=4
  RollBias V : Inport  Port=5
  PitchBias V (right) : Inport  Port=6
  a2 : Inport  Port=7
  Bias_v : Inport  Port=8
  Phase (deg) : Inport  Port=9
  In1 : Inport  Port=10
  MATLAB Function : MATLAB Function  TreatAsAtomicUnit=on  VariantControl=Choice_1
  Terminator : Terminator
  signal generator a3 : Subsystem
  X (m) : Outport
  Y (m) : Outport  Port=2
  Z (m) : Outport  Port=3
  alpha (radians) : Outport  Port=4
  beta (radians) : Outport  Port=5
  gamma (radians) : Outport  Port=6
  wires:
  ? -> MATLAB Function/6(port)
  signal generator a3/1(Bias_D2A) -> MATLAB Function/2(left_voltage_v)
  ? -> MATLAB Function/1(dt_s)
  signal generator a3/3(D2A DriveSignal 2) -> MATLAB Function/4(bias_voltage_v)
  signal generator a3/2(D2A DriveSignal 1) -> MATLAB Function/3(right_voltage_v)
  ? -> MATLAB Function/5(host)
  a2/1 -> signal generator a3/9(a2)
  PitchBias V (left)/1 -> signal generator a3/5(PitchBias V (left))
  Amplitude/1 -> signal generator a3/4(Amplitude)
  Bias_v/1 -> signal generator a3/2(Bias_v)
  PitchBias V (right)/1 -> signal generator a3/8(PitchBias V (right))
  RollBias V/1 -> signal generator a3/6(RollBias V)
  Phase (deg)/1 -> signal generator a3/7(Phase (deg))
  frequency (hz)/1 -> signal generator a3/3(frequency (hz))
  EnableSignal/1 -> signal generator a3/1(EnableSignal)
  In1/1 -> Terminator/1
  MATLAB Function/1(x) -> X (m)/1
  MATLAB Function/2(y) -> Y (m)/1
  MATLAB Function/3(z) -> Z (m)/1
  MATLAB Function/4(alpha_rad) -> alpha (radians)/1
  MATLAB Function/5(beta_rad) -> beta (radians)/1
  MATLAB Function/6(gamma_rad) -> gamma (radians)/1

== system updated_target_driver_2026/Vicon Post Processing1/Raw rotation matrix ==
  alpha : Inport
  beta : Inport  Port=2
  gamma : Inport  Port=3
  Mux : Mux  Inputs=9
  Rotation Matrix : Subsystem
  R : Outport
  wires:
  alpha/1 -> Rotation Matrix/1(alpha)
  beta/1 -> Rotation Matrix/2(beta)
  gamma/1 -> Rotation Matrix/3(gamma)
  Mux/1 -> R/1
  Rotation Matrix/1(R11) -> Mux/1
  Rotation Matrix/2(R12) -> Mux/2
  Rotation Matrix/3(R13) -> Mux/3
  Rotation Matrix/4(R21) -> Mux/4
  Rotation Matrix/5(R22) -> Mux/5
  Rotation Matrix/6(R23) -> Mux/6
  Rotation Matrix/7(R31) -> Mux/7
  Rotation Matrix/8(R32) -> Mux/8
  Rotation Matrix/9(R33) -> Mux/9

== system updated_target_driver_2026/Vicon Post Processing1/Vicon Validity check ==
  "Rotation Matrix " : Inport
  Compare To Zero2 : simulink/Logic and Bit Operations/Compare To Zero  relop===  OutDataTypeStr=uint8
  Constant : Constant
  Data Type Conversion1 : DataTypeConversion  OutDataTypeStr=double  SaturateOnIntegerOverflow=off  RndMeth=Floor
  Delay : Delay  DelayLength=1  InitialCondition=0
  Delay2 : Delay  DelayLength=1  InitialCondition=0
  MATLAB Function3 : MATLAB Function  TreatAsAtomicUnit=on
  SaturatingRamp : DiscreteIntegrator  gainval=sampling_f  ExternalReset=falling  SampleTime=-1  UpperSaturationLimit=1  LowerSaturationLimit=0  ICPrevOutput=DiscIntNeverNeededParam  ICPrevScaledInput=DiscIntNeverNeededParam
  type conv : DataTypeConversion  OutDataTypeStr=double  SaturateOnIntegerOverflow=off  RndMeth=Floor
  "Vicon Update flag " : Outport
  Vicon Count : Outport  Port=2
  wires:
  Data Type Conversion1/1 -> Delay2/1, "Vicon Update flag "/1
  Delay/1 -> MATLAB Function3/1(R_prev)
  SaturatingRamp/1 -> Data Type Conversion1/1
  type conv/1 -> SaturatingRamp/2
  MATLAB Function3/1(y) -> Compare To Zero2/1
  Constant/1 -> SaturatingRamp/1
  Compare To Zero2/1 -> type conv/1
  "Rotation Matrix "/1 -> MATLAB Function3/2(R_cur), Delay/1
  Delay2/1 -> Vicon Count/1

== system updated_target_driver_2026/Desired attitude and normalized error/Geometric derivative for Rd in SO(3)/filtered derivative1 ==
  In1 : Inport
  low pass3 : DiscreteTransferFcn  Numerator=vlp_num  Denominator=vlp_den
  Out1 : Outport
  wires:
  low pass3/1 -> Out1/1
  In1/1 -> low pass3/1

== system updated_target_driver_2026/Desired attitude and normalized error/Geometric derivative for Rd in SO(3)/filtered derivative5 ==
  In1 : Inport
  low pass3 : DiscreteTransferFcn  Numerator=lp_num  Denominator=lp_den
  Out1 : Outport
  wires:
  low pass3/1 -> Out1/1
  In1/1 -> low pass3/1

== system updated_target_driver_2026/Desired attitude and normalized error/saturated normalized error observation/Saturated angular velocity eOmega  ==
  omega : Inport
  "omega_desired " : Inport  Port=2
  R_cur : Inport  Port=3
  R_desired : Inport  Port=4
  Compute attitude error eR : MATLAB Function  TreatAsAtomicUnit=on
  Demux1 : Demux  Outputs=3
  Gain : Gain  Gain=2/(upp_bound-low_bound)
  Gain1 : Gain  Gain=2/(upp_bound-low_bound)
  Gain2 : Gain  Gain=2/(upp_bound-low_bound)
  Mux5 : Mux  Inputs=3
  Saturation1 : Saturate  UpperLimit=upp_bound  LowerLimit=low_bound
  Saturation2 : Saturate  UpperLimit=upp_bound  LowerLimit=low_bound
  Saturation3 : Saturate  UpperLimit=upp_bound  LowerLimit=low_bound
  Normalized angular velocity : Outport
  wires:
  Saturation1/1 -> Gain/1
  Mux5/1 -> Normalized angular velocity/1
  Saturation2/1 -> Gain1/1
  Gain/1 -> Mux5/1
  Gain1/1 -> Mux5/2
  "omega_desired "/1 -> Compute attitude error eR/4(omega_desired)
  Demux1/1 -> Saturation1/1
  R_desired/1 -> Compute attitude error eR/2(R_desired)
  R_cur/1 -> Compute attitude error eR/1(R_cur)
  omega/1 -> Compute attitude error eR/3(omega)
  Compute attitude error eR/1(y) -> Demux1/1
  Demux1/2 -> Saturation2/1
  Demux1/3 -> Saturation3/1
  Saturation3/1 -> Gain2/1
  Gain2/1 -> Mux5/3

== system updated_target_driver_2026/Desired attitude and normalized error/saturated normalized error observation/Saturated normalized eR ==
  Current averaged rotation M : Inport
  R_desired : Inport  Port=2
  Compute attitude error eR : MATLAB Function  TreatAsAtomicUnit=on
  Gain6 : Gain  Gain=2/(upp_bound_eR-low_bound_eR)
  Saturation4 : Saturate  UpperLimit=upp_bound_eR  LowerLimit=low_bound_eR
  normalized eR : Outport
  wires:
  Compute attitude error eR/1(y) -> Saturation4/1
  Saturation4/1 -> Gain6/1
  R_desired/1 -> Compute attitude error eR/2(R_desired)
  Gain6/1 -> normalized eR/1
  Current averaged rotation M/1 -> Compute attitude error eR/1(R_cur)

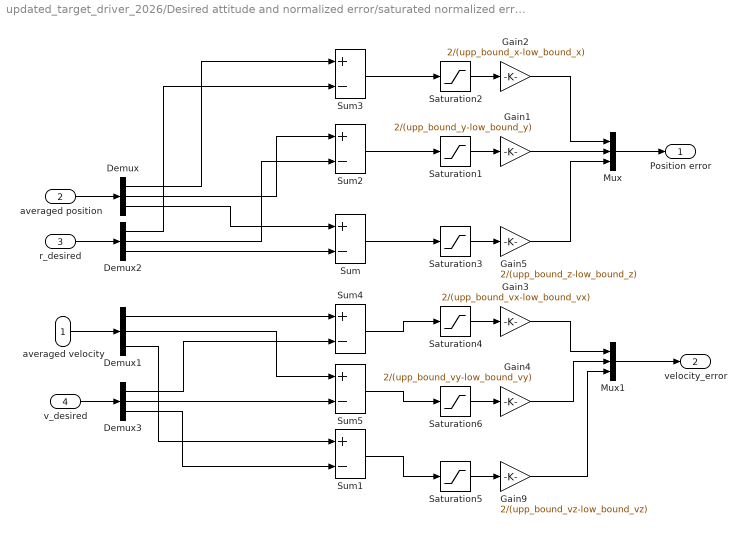
== system updated_target_driver_2026/Desired attitude and normalized error/saturated normalized error observation/saturated normalized altitude error  ==
  averaged velocity : Inport
  averaged position : Inport  Port=2
  "r_desired " : Inport  Port=3
  v_desired : Inport  Port=4
  Demux{,1..3} (4 alike) : Demux  Outputs=3
  Gain1 : Gain  Gain=2/(upp_bound_y-low_bound_y)
  Gain2 : Gain  Gain=2/(upp_bound_x-low_bound_x)
  Gain3 : Gain  Gain=2/(upp_bound_vx-low_bound_vx)
  Gain4 : Gain  Gain=2/(upp_bound_vy-low_bound_vy)
  Gain5 : Gain  Gain=2/(upp_bound_z-low_bound_z)
  Gain9 : Gain  Gain=2/(upp_bound_vz-low_bound_vz)
  Mux : Mux  Inputs=3
  Mux1 : Mux  Inputs=3
  Saturation1 : Saturate  UpperLimit=upp_bound_y  LowerLimit=low_bound_y
  Saturation2 : Saturate  UpperLimit=upp_bound_x  LowerLimit=low_bound_x
  Saturation3 : Saturate  UpperLimit=upp_bound_z  LowerLimit=low_bound_z
  Saturation4 : Saturate  UpperLimit=upp_bound_vx  LowerLimit=low_bound_vx
  Saturation5 : Saturate  UpperLimit=upp_bound_vz  LowerLimit=low_bound_vz
  Saturation6 : Saturate  UpperLimit=upp_bound_vy  LowerLimit=low_bound_vy
  Sum{,1..5} (6 alike) : Sum  Inputs=+-
  Position error : Outport
  velocity_error : Outport  Port=2
  wires:
  Demux2/3 -> Sum/2
  Sum/1 -> Saturation3/1
  Sum1/1 -> Saturation5/1
  Gain5/1 -> Mux/3
  Saturation3/1 -> Gain5/1
  Saturation5/1 -> Gain9/1
  Gain9/1 -> Mux1/3
  Mux1/1 -> velocity_error/1
  averaged velocity/1 -> Demux1/1
  averaged position/1 -> Demux/1
  Demux/3 -> Sum/1
  Demux1/3 -> Sum1/1
  "r_desired "/1 -> Demux2/1
  Saturation1/1 -> Gain1/1
  Sum2/1 -> Saturation1/1
  Demux2/2 -> Sum2/2
  Demux/2 -> Sum2/1
  Sum3/1 -> Saturation2/1
  Saturation2/1 -> Gain2/1
  Demux/1 -> Sum3/1
  Demux2/1 -> Sum3/2
  v_desired/1 -> Demux3/1
  Demux3/3 -> Sum1/2
  Saturation4/1 -> Gain3/1
  Gain3/1 -> Mux1/1
  Sum4/1 -> Saturation4/1
  Demux3/1 -> Sum4/2
  Demux1/1 -> Sum4/1
  Saturation6/1 -> Gain4/1
  Gain4/1 -> Mux1/2
  Sum5/1 -> Saturation6/1
  Demux3/2 -> Sum5/2
  Demux1/2 -> Sum5/1
  Gain2/1 -> Mux/1
  Gain1/1 -> Mux/2
  Mux/1 -> Position error/1

== system updated_target_driver_2026/Observer for averaged system1/Attitude Observer/Geometric Averaging Rotation Matix ==
  note: Geometric mean in SO(3)
      | 1) Output the Geometric average over one cycle (n=4 samples: 500Hz vicon sampling and 160Hz flapping signal)
      |
      | Patrick 2021 Mar
  Vicon Update flag : Inport
  Current Rotation : Inport  Port=2
  Averaged quaternion : MATLAB Function  TreatAsAtomicUnit=on
  Delay6 : Delay  DelayLength=1  InitialCondition=0
  Demux3 : Demux
  Demux4 : Demux
  Geometric Averaging Rotation M : Subsystem
  Mux3 : Mux
  Mux4 : Mux
  Raw quaternion : MATLAB Function  TreatAsAtomicUnit=on
  Averaged quaternion output : Outport
  "Averaged Rotation Matrix " : Outport  Port=2
  "Raw quaternion output " : Outport  Port=3
  Previous Averaged Rotation Matrix : Outport  Port=4
  wires:
  Raw quaternion/1(quat) -> Demux4/1
  Demux4/3 -> Mux4/3
  Demux4/4 -> Mux4/4
  Demux4/1 -> Mux4/1
  Demux4/2 -> Mux4/2
  Mux4/1 -> "Raw quaternion output "/1
  Vicon Update flag/1 -> Geometric Averaging Rotation M/2(Vicon Update)
  Current Rotation/1 -> Raw quaternion/1(R), Geometric Averaging Rotation M/1("Current Rotation ")
  Mux3/1 -> Averaged quaternion output/1
  Demux3/4 -> Mux3/4
  Averaged quaternion/1(quat) -> Demux3/1
  Demux3/3 -> Mux3/3
  Geometric Averaging Rotation M/1(Averaged Rotation Matrix) -> Delay6/1, Averaged quaternion/1(R), "Averaged Rotation Matrix "/1
  Demux3/2 -> Mux3/2
  Demux3/1 -> Mux3/1
  Delay6/1 -> Geometric Averaging Rotation M/3("Previous Averaged Rotation "), Previous Averaged Rotation Matrix/1

== system updated_target_driver_2026/Observer for averaged system1/Attitude Observer/Geometric derivative in SO(3) ==
  note: First order geometric derivative in SO(3)
      | Patrick 2021 Mar
  Previous Averaged Rotation M : Inport
  Vicon Count : Inport  Port=2
  Current Averaged Rotation M : Inport  Port=3
  "Vicon Update Flag " : Inport  Port=4
  Demux2 : Demux  Outputs=3
  "First order geometric derivative in SO(3) " : MATLAB Function  TreatAsAtomicUnit=on
  Mux2 : Mux  Inputs=3
  Previous Omega : Delay  DelayLength=1  InitialCondition=0
  filtered derivative5 : Subsystem
  Filtered Geometric derivative in SO(3) : Outport
  wires:
  Previous Omega/1 -> "First order geometric derivative in SO(3) "/3(omega_prev)
  Previous Averaged Rotation M/1 -> "First order geometric derivative in SO(3) "/1(R_prev)
  Demux2/1 -> Mux2/1
  Demux2/2 -> Mux2/2
  filtered derivative5/1(Out1) -> Demux2/1
  Mux2/1 -> Filtered Geometric derivative in SO(3)/1
  "First order geometric derivative in SO(3) "/1(omega) -> Previous Omega/1, filtered derivative5/1(In1)
  Demux2/3 -> Mux2/3
  "Vicon Update Flag "/1 -> "First order geometric derivative in SO(3) "/4(update)
  Current Averaged Rotation M/1 -> "First order geometric derivative in SO(3) "/2(R_cur)
  Vicon Count/1 -> "First order geometric derivative in SO(3) "/5(count)

== system updated_target_driver_2026/Observer for averaged system1/Euler derivative & filtered angular velocity /filtered derivative ==
  In1 : Inport
  att_s : Gain  Gain=att_s
  filtered derivative : simulink/Discrete/Transfer Fcn Lead or Lag  PoleZ=k_da  ZeroZ=1  ICPrevOutput=0.0  ICPrevInput=0.0  DoSatur=off
  low pass3 : DiscreteTransferFcn  Numerator=lp_num  Denominator=lp_den
  Out1 : Outport
  wires:
  att_s/1 -> filtered derivative/1
  In1/1 -> att_s/1
  low pass3/1 -> Out1/1
  filtered derivative/1 -> low pass3/1

== system updated_target_driver_2026/Observer for averaged system1/Position Observer/LowPassFiltere1 ==
  In1 : Inport
  low pass3 : DiscreteTransferFcn  Numerator=lp_num  Denominator=lp_den
  Out1 : Outport
  wires:
  low pass3/1 -> Out1/1
  In1/1 -> low pass3/1

== system updated_target_driver_2026/Observer for averaged system1/Position Observer/LowPassFiltere2 ==
  In1 : Inport
  low pass3 : DiscreteTransferFcn  Numerator=lp_num  Denominator=lp_den
  Out1 : Outport
  wires:
  low pass3/1 -> Out1/1
  In1/1 -> low pass3/1

== system updated_target_driver_2026/Plant/signal generator a3/Bias_Signal ==
  note: time constant = 0.002sec
  QuasiEnable : Inport
  BiasVolts : Inport  Port=2
  AveragedBias : Subsystem
  PreGain : Gain
  Product : Product  RndMeth=Zero
  SIgnalForRamp_binary : Subsystem
  SaturatingRamp : DiscreteIntegrator  gainval=10  SampleTime=-1  LimitOutput=on  UpperSaturationLimit=1  LowerSaturationLimit=0  ICPrevOutput=DiscIntNeverNeededParam  ICPrevScaledInput=DiscIntNeverNeededParam
  BiasD2A : Outport
  wires:
  PreGain/1 -> BiasD2A/1
  BiasVolts/1 -> AveragedBias/1(In1)
  QuasiEnable/1 -> SIgnalForRamp_binary/1(In1)
  SIgnalForRamp_binary/1(Out1) -> SaturatingRamp/1
  SaturatingRamp/1 -> Product/1
  AveragedBias/1(Out1) -> Product/2
  Product/1 -> PreGain/1

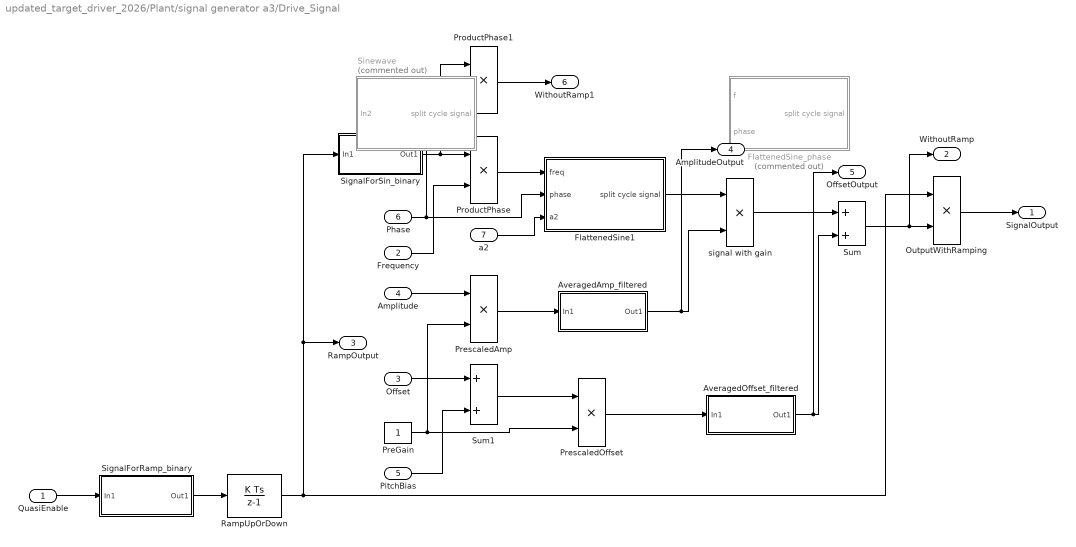
== system updated_target_driver_2026/Plant/signal generator a3/Drive_Signal ==
  QuasiEnable : Inport
  Frequency : Inport  Port=2
  Offset : Inport  Port=3
  Amplitude : Inport  Port=4
  PitchBias : Inport  Port=5
  Phase : Inport  Port=6
  "a2 " : Inport  Port=7
  AveragedAmp_filtered : Subsystem
  AveragedOffset_filtered : Subsystem
  FlattenedSine1 : Subsystem
  FlattenedSine_phase : Subsystem  Commented=on
  OutputWithRamping : Product  RndMeth=Zero
  PreGain : Constant
  PrescaledAmp : Product  RndMeth=Zero
  PrescaledOffset : Product  RndMeth=Zero
  ProductPhase : Product  RndMeth=Zero
  ProductPhase1 : Product  RndMeth=Zero
  RampUpOrDown : DiscreteIntegrator  gainval=10  SampleTime=-1  LimitOutput=on  UpperSaturationLimit=1  LowerSaturationLimit=0  ICPrevOutput=DiscIntNeverNeededParam  ICPrevScaledInput=DiscIntNeverNeededParam
  SignalForRamp_binary : Subsystem
  SignalForSin_binary : Subsystem
  Sinewave : Subsystem  Commented=on
  Sum : Sum
  Sum1 : Sum
  signal with gain : Product  RndMeth=Zero
  SignalOutput : Outport
  WithoutRamp : Outport  Port=2
  RampOutput : Outport  Port=3
  AmplitudeOutput : Outport  Port=4
  OffsetOutput : Outport  Port=5
  WithoutRamp1 : Outport  Port=6
  wires:
  OutputWithRamping/1 -> SignalOutput/1
  Sum/1 -> WithoutRamp/1, OutputWithRamping/2
  PrescaledOffset/1 -> AveragedOffset_filtered/1(In1)
  AveragedAmp_filtered/1(Out1) -> AmplitudeOutput/1, signal with gain/2
  PrescaledAmp/1 -> AveragedAmp_filtered/1(In1)
  "a2 "/1 -> FlattenedSine1/3(a2)
  ProductPhase/1 -> FlattenedSine1/1(freq)
  ProductPhase1/1 -> WithoutRamp1/1
  Offset/1 -> Sum1/1
  AveragedOffset_filtered/1(Out1) -> OffsetOutput/1, Sum/2
  signal with gain/1 -> Sum/1
  SignalForSin_binary/1(Out1) -> ProductPhase1/1, ProductPhase/1
  Amplitude/1 -> PrescaledAmp/1
  Sum1/1 -> PrescaledOffset/1
  Frequency/1 -> ProductPhase/2
  PreGain/1 -> PrescaledAmp/2, PrescaledOffset/2
  FlattenedSine1/1(split cycle signal) -> signal with gain/1
  QuasiEnable/1 -> SignalForRamp_binary/1(In1)
  SignalForRamp_binary/1(Out1) -> RampUpOrDown/1
  Phase/1 -> ProductPhase1/2, FlattenedSine1/2(phase)
  PitchBias/1 -> Sum1/2
  RampUpOrDown/1 -> SignalForSin_binary/1(In1), RampOutput/1, OutputWithRamping/1
